simulink model "LQR_bloques_SS_LQR_cascada_PID_controller_NonLinear"  (R2023a)
settings: Solver=VariableStepAuto  StartTime=0.0  StopTime=t_sim  RelTol=1e-1
undefined symbols (not defined in the file): A, A_model, A_motor, B, B_mag0, B_model2, B_motor, C_model2, C_motor, D_motor, DeltaH_error_Gain, Error_ref_Gain, Gamma, I, J, K3_2, K4_2, K_gamma, Ke, Kt, La, Mgt_power_Gain, n_cal, omegaZ_inicial, R_mgt, Ra, RW_omega_max, RW_power_Gain, T_ext, T_max, T_max_mgt
libraries: simulink_extras x7, matrix_library x5, vrlib x2, slpidlib x2, aerolibutil x1, simulink x1
(part 1 of 2)
settings Model: Creator=Personal  LastModifiedBy=Personal
settings SolverCC: ZeroCrossAlgorithm=Adaptive
settings DebuggingCC: MaskedZcDiagnostic=none  IgnoredZcDiagnostic=none

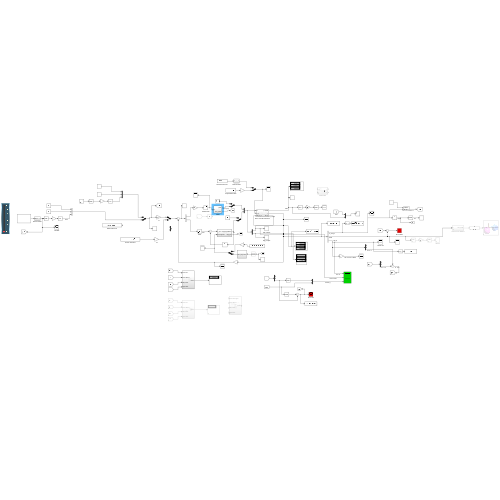
[thumbnail: Simulink's stored preview of the top-level diagram]
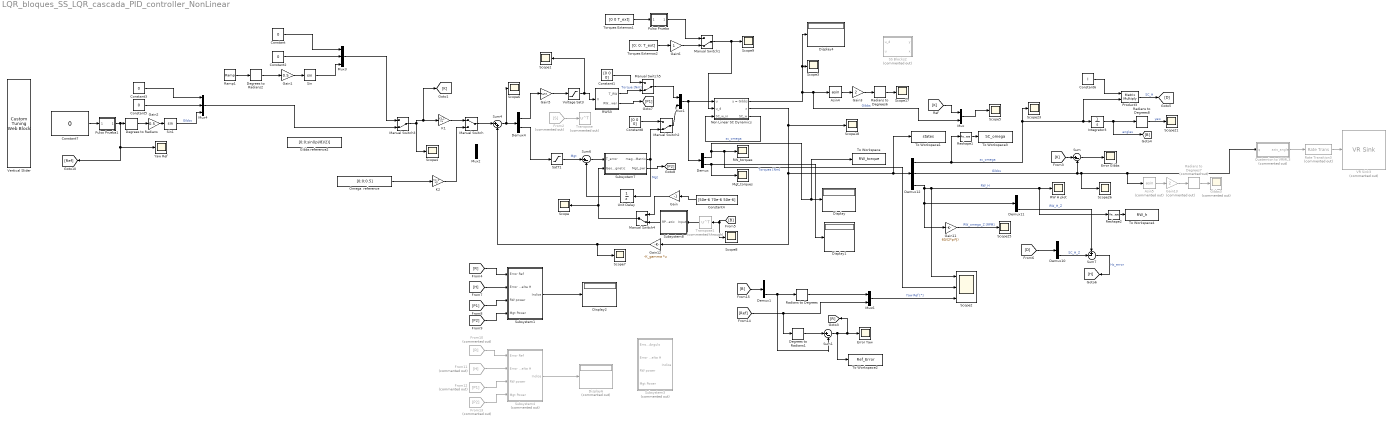
== system LQR_bloques_SS_LQR_cascada_PID_controller_NonLinear ==
  Asin4 : Trigonometry  Operator=asin
  Asin5 : Trigonometry  Commented=on  Operator=asin
  Constant{,2..3,5,7} (5 alike) : Constant  Value=0
  Constant1 : Constant  Value=[0 0 0]
  Constant4 : Constant  Value=[50e-6 70e-6 50e-6]
  Constant6 : Constant  Value=I
  Constant8 : Constant  Value=[0 0 0]
  Degrees to Radians : simulink_extras/Transformations/Degrees to Radians
  Degrees to Radians1 : simulink_extras/Transformations/Degrees to Radians
  Degrees to Radians2 : simulink_extras/Transformations/Degrees to Radians
  Demux : Demux  Outputs=2
  Demux{1,10..12} (4 alike) : Demux  Outputs=3
  Demux4 : Demux  Outputs=2
  Display{,1..2,4} (4 alike) : Display
  Display6 : Display  Commented=on
  Error Gibbs : Scope
  Error Yaw : Scope
  From10 : From  Commented=on  GotoTag=R
  From11 : From  Commented=on  GotoTag=H
  From12 : From  Commented=on  GotoTag=P1
  From13 : From  Commented=on  GotoTag=P2
  From2 : From  Commented=on  GotoTag=S
  Gain : Gain  Gain=-1
  Gain1 : Gain  Gain=0.5
  Gain11 : Gain  Gain=60/(2*pi*J)
  Gain12 : Gain  Gain=-K_gamma  Multiplication=Matrix(K*u)
  Gain13 : Gain  Commented=on  Gain=2
  Gain2 : Gain  Gain=0.5
  Gain3 : Gain  Gain=2
  Gain5 : Gain  Gain=Ra/Kt
  Gain6 : Gain
  Gibbs reference2 : Constant  Value=[0;0;sin((pi/8)/2)]  VectorParams1D=off
  Gibbs3 : Scope  Commented=on
  Integrator3 : Integrator  InitialCondition=[0;0;0]
  K1 : Gain  Gain=K3_2  Multiplication=Matrix(K*u)
  K2 : Gain  Gain=K4_2  Multiplication=Matrix(K*u)
  Manual Switch : ManualSwitch
  Manual Switch{1..5} (5 alike) : ManualSwitch  CurrentSetting=0
  Mgt_torques : Scope
  Mux{,1..2,6} (4 alike) : Mux  Inputs=2
  Mux3 : Mux  Inputs=3
  Mux4 : Mux  Inputs=3
  Non Linear SC Dynamics : Subsystem
  Omega  reference : Constant  Value=[0;0;0.5]
  Product3 : Product  Multiplication=Matrix(*)
  Pulso Prueba : Subsystem
  Pulso Prueba1 : Subsystem
  Quaternion to VRML3 : Subsystem  Commented=on
  RW H plot : Scope
  RWS3 : Subsystem
  RW_torques : Scope
  Radians to Degrees : simulink_extras/Transformations/Radians to Degrees
  Radians to Degrees6 : simulink_extras/Transformations/Radians to Degrees
  Radians to Degrees7 : simulink_extras/Transformations/Radians to Degrees  Commented=on
  Radians to Degrees8 : simulink_extras/Transformations/Radians to Degrees
  Ramp1 : simulink/Sources/Ramp  slope=0.5  start=0  InitialOutput=0
  Rate Transition3 : RateTransition  Commented=on
  Reshape1 : Reshape
  Reshape2 : Reshape
  SS Blocks2 : Subsystem  Commented=on
  SatT1 : Saturate  UpperLimit=T_max_mgt  LowerLimit=-T_max_mgt
  Scope{,1,3..9,17..18,21,23,25..26} (15 alike) : Scope
  Scope2 : Scope  NumInputPorts=3
  Sin : Trigonometry
  Sin1 : Trigonometry
  Subsystem1 : Subsystem
  Subsystem3 : Subsystem  Commented=on
  Subsystem4 : Subsystem  Commented=on
  Subsystem7 : Subsystem
  Subsystem8 : Subsystem
  Sum : Sum  Inputs=|+-
  Sum1 : Sum  Inputs=|+-
  Sum4 : Sum  Inputs=|++
  Sum6 : Sum  Inputs=|+-
  Sum7 : Sum  Inputs=+-|
  To Workspace : ToWorkspace  VariableName=RW_torque  SaveFormat=Structure With Time  SampleTime=-1
  To Workspace1 : ToWorkspace  VariableName=states  SaveFormat=Structure With Time  SampleTime=-1
  To Workspace2 : ToWorkspace  VariableName=Ref_Error  SaveFormat=Structure With Time  SampleTime=-1
  To Workspace3 : ToWorkspace  VariableName=SC_omega  SaveFormat=Structure With Time  SampleTime=-1
  To Workspace4 : ToWorkspace  VariableName=RW_h  SaveFormat=Structure With Time  SampleTime=-1
  Torques Externos1 : Constant  Value=[0 0 T_ext]
  Torques Externos2 : Constant  Value=[0; 0; T_ext]
  Transpose : Math  Commented=on  Operator=transpose
  Transpose1 : Math  Commented=through  Operator=transpose
  Unit Delay : UnitDelay  SampleTime=-1  HasFrameUpgradeWarning=on
  VR Sink3 : vrlib/VR Sink  Commented=on  InstantiateOnLoad=on  SampleTime=0.1  ViewEnable=on  RemoteChange=off  RemoteView=off  FieldsWritten=STLB_Transform.rotation.4.1.1.double  WorldFileName=EscenarioCubeSat.x3d  AutoView=off  VideoDimensions=[]  AllowVariableSize=off
  Vertical Slider : CustomTuningWebBlock  LabelPosition=Hide  ShowInitialText=on  Configuration="{\"components\":[{\"name\":\"LinearScaleComponent\",\"settings\":{\"bounds\":{\"max\":360,\"min\":0,\"tickInterval\":\"auto\"},\"internalTickHeightScaleFactor\":0.5,\"labelColor\":[255,255,200],\"labelFont\":{\"font\":\"Arial\",\"fontSize\":12},\"labelOffset\":0.05,\"labelTransparency\":1,\"needleImage\":{\"size\":[596,842],\"src\":\"data:image\\/svg+xml;base64,PD94bWwgdmVyc2lvbj0iMS4wIiBlbmNvZGluZz0idXRmLTgiPz4NCjwhLS0gR2VuZXJhdG9yOiBBZG9iZSBJbGx1c3RyYXRvciAyNS4wLjAsIFNWRyBFeHBvcnQgUGx1Zy1JbiAuIFNWRyBWZXJzaW9uOiA2LjAwIEJ1aWxkIDApICAtLT4NCjxzdmcgdmVyc2lvbj0iMS4xIg0KCSBpZD0ic3ZnOCIgeG1sbnM6Y2M9Imh0dHA6Ly9jcmVhdGl2ZWNvbW1vbnMub3JnL25zIyIgeG1sbnM6ZGM9Imh0dHA6Ly9wdXJsLm9yZy9kYy9lbGVtZW50cy8xLjEvIiB4bWxuczppbmtzY2FwZT0iaHR0cDovL3d3dy5pbmtzY2FwZS5vcmcvbmFtZXNw ...(+2420 chars)\",\"srcOrientation\":\"horizontal\"},\"needleOffset\":[0.0642123287671233,-0.8044596912521441],\"needleSize\":{\"height\":0.07668067226890757,\"width\":0.4337797619047619},\"position\":[0.03623949579831933,0.2829861111111111,0.6088789682539683,0.9196428571428571],\"referencePoint\":\"auto\",\"scaleColors\":[],\"scaleColorsSize\":0.2,\"scaleDirection\":\"BT\",\"showLabels\":1,\"showMinorTicks\":0,\"showSpanLine\":1,\"showTicks\":1,\"tickColor\":[252,252,197],\"tickTransparency\":1,\"valueBarColor\":[0,114,189],\"valueBarOffset\":-0.27,\"valueBarSize\":0.1,\"valueBarTransparency\":1}},{\"name\":\"BackgroundImageComponent\",\"settings\":{\"image\":{\"size\":[380,101],\"src\":\"data:image\\/svg+xml;base64,PHN2ZyB4bWxucz0iaHR0cDovL3d3dy53My5vcmcvMjAwMC9zdmciIHhtbG5zOnhsaW5rPSJodHRwOi8vd3d3LnczLm9yZy8xOTk5L3hsaW5rIiB2aWV3Qm94PSIwIDAgMzgwIDEwMSI+PGRlZnM+PHN0eWxlPi5jbHMtMXtmaWxsOiMwMDJiNDI7fS5jbHMtMntmaWxsOiM0MjcwODI7fS5jbHMtM3tmaWxsOnVybCgjcmFkaWFsLWdyYWRpZW50KTt9LmNscy00e2ZpbGw6I2M4YzhjODtzdHJva2U6IzAwMDt9PC9zdHlsZT48cmFkaWFsR3JhZGllbnQgaWQ9InJhZGlhbC1ncmFkaWVudCIgY3g9IjE5MCIgY3k9IjUwLjUiIHI9IjI2OS4yMSIgZ3JhZGllbnRVbml0cz0idXNlclNwYWNlT25Vc2UiPjxzdG9wIG9mZnNldD0iMC4wMSIgc3RvcC1jb2xvcj0iIzNlNGY1OCIvPjxzdG9wIG9mZnNldD0iMC4wNiIgc3RvcC1jb2xvcj0iIzQ0NTc2MSIvPjxzdG9wIG9mZnNldD0iMC4xNSIgc3RvcC1jb2xvcj0iIzU1NmE3NiIvPjxzdG9wIG9mZnNldD0iMC4yNSIgc3RvcC1jb2xvcj0iIzZkODg5NSIvPjxzdG9wIG9mZnNldD0iMC4zOCIgc3RvcC1jb2xvcj0iIzhmYjJjMyIvPjxzdG9wIG9mZnNldD0iMC41MiIgc3RvcC1jb2xvcj0iI2I2ZTRmYSIvPjxzdG9wIG9mZnNldD0iMSIgc3RvcC1jb2xvcj0iIzE1NDY1NyIvPjwvcmFkaWFsR3JhZGllbnQ+PC9kZWZzPjxnIGlkPSJmcmFtZSI+PGcgaWQ9IkxheWVyXzIiIGRhdGEtbmFtZT0iTGF5ZXIgMiI+PGcgaWQ9IkxheWVyXzEtMiIgZGF0YS1uYW1lPSJMYXllciAxLTIiPjxyZWN0IGlkPSJyZWN0MTAzNiIgY2xhc3M9ImNscy0xIiB4PSIxMSIgeT0iMTEiIHdpZHRoPSIzNTgiIGhlaWdodD0iNzkiLz48cGF0aCBpZD0icGF0aDEwMzgiIGNsYXNzPSJjbHMtMiIgZD0iTTgsOFY5M0gzNzJWOFpNMzY5LDkwSDExVjExSDM2OVoiLz48cGF0aCBpZD0icGF0aDEwNDAiIGNsYXNzPSJjbHMtMyIgZD0iTTAsMFYxMDFIMzgwVjBaTTM3Miw5M0g4VjhIMzcyWiIvPjwvZz48L2c+PC9nPjxnIGlkPSJ0cmFjayI+PHBhdGggaWQ9InJlY3QxNjExIiBjbGFzcz0iY2xzLTQiIGQ9Ik0zMy4zNywyNi41OUgzNDYuNjNjNCwwLDcuMjUsMi42LDcuMjUsNS44MWgwYzAsMy4yMS0zLjI1LDUuODItNy4yNSw1LjgySDMzLjM3Yy00LDAtNy4yNS0yLjYxLTcuMjUtNS44MmgwQzI2LjEyLDI5LjE5LDI5LjM3LDI2LjU5LDMzLjM3LDI2LjU5WiIvPjwvZz48L3N2Zz4=\",\"srcOrientation\":\"horizontal\"},\"position\":[0,0,1,1],\"scaleMode\":\"0\"}},{\"name\":\"ForegroundImageComponent\",\"settings\":{\"image\":{\"size\":[0,0],\"src\":\"default\",\"srcOrientation\":[]},\"isForeground\":1,\"position\":[0,0,1,1],\"scaleMode\":\"0\"}}],\"settings\":{\"BindingType\":\"param\",\"aspectRatio\":3.7777777777777777,\"backgroundColor\":[0,0,0,\"1\"],\"backgroundOffset\":0,\"backgroundOpacity\":1,\"fixedAspectRatio\":\"on\",\"foregroundColor\":[252,252,196],\"orientation\":\"vertical\",\"showBackgroundColor\":false,\"value\":0,\"version\":\"R2023a\"},\"type\":\"LinearGauge\"}"
  Voltage Sat3 : Saturate  UpperLimit=6  LowerLimit=-6
  Yaw Ref : Scope
  wires:
  K1/1 -> Manual Switch/1
  Mux1/1 -> Non Linear SC Dynamics/1(u), Demux/1
  Gain3/1 -> Radians to Degrees6/1
  Non Linear SC Dynamics/1(y = Gibbs) -> Display4/1, Scope3/1, Mux/2, Asin4/1  "Gibbs"
  Asin4/1 -> Gain3/1
  Radians to Degrees6/1 -> Scope17/1
  Demux/1 -> To Workspace/1, Display/1, Scope2/2, RW_torques/1  "Torques [Nm]"
  Demux/2 -> Display1/1, Mgt_torques/1
  Voltage Sat3/1 -> Scope1/1, RWS3/1(V)
  Gain5/1 -> Voltage Sat3/1
  SatT1/1 -> Sum6/1  "Mgt"
  Sum6/1 -> Subsystem7/1(T_error)
  Manual Switch4/1 -> Subsystem7/2(Geomagnetic), Scope/1
  Demux4/1 -> Gain5/1
  Demux4/2 -> SatT1/1
  Gain12/1 -> Scope7/1, Sum4/2
  Sum4/1 -> Scope6/1, Demux4/1
  Subsystem7/1(magTorqueMatrix) -> Unit Delay/1, Manual Switch2/2  "Mgt"
  RWS3/1(T_RW) -> Manual Switch5/2  "Torque [Nm]"
  Constant4/1 -> Gain/1
  Subsystem8/1(RPY_Magnetic) -> Manual Switch4/2
  Transpose1/1 -> Subsystem8/1(Input)
  Gain/1 -> Manual Switch4/1
  [D] -> Demux10/1
  Non Linear SC Dynamics/2(x) -> Gain12/1, To Workspace1/1, Demux12/1, Scope18/1
  Radians to Degrees7/1 -> Gibbs3/1
  Demux10/3 -> Sum7/2  "SC_H_Z"
  Radians to Degrees8/1 -> Scope21/1  "yaw"
  Demux11/3 -> Sum7/1  "RW_H_Z"
  Rate Transition3/1 -> VR Sink3/1
  Quaternion to VRML3/1(axis_angle) -> Rate Transition3/1
  Gain13/1 -> Radians to Degrees7/1
  Product3/1 -> [D]  "SC_H"
  Integrator3/1 -> [B], Radians to Degrees8/1  "angles"
  Gain11/1 -> Scope25/1  "RW_omega_Z [RPM]"
  Demux12/2 -> Asin5/1, Quaternion to VRML3/1(q), Scope26/1, Sum/2  "Gibbs"
  Sum7/1 -> [H]  "Hz_error"
  Asin5/1 -> Gain13/1
  Constant6/1 -> Product3/1
  Demux12/3 -> Scope2/1, Reshape2/1, RW H plot/1, Gain11/1, Demux11/1  "RW_H"
  Demux12/1 -> Integrator3/1, Product3/2, Scope23/1, Reshape1/1  "sc_omega"
  [B] -> Scope8/1, Transpose1/1
  Unit Delay/1 -> Sum6/2
  Omega  reference/1 -> K2/1
  Manual Switch/1 -> Sum4/1
  K2/1 -> Manual Switch/2
  Torques Externos2/1 -> Gain6/1
  Manual Switch2/1 -> Mux1/2
  Manual Switch3/1 -> Scope4/1, K1/1, [K]
  Mux/1 -> Scope5/1
  [K] -> Mux/1
  Manual Switch5/1 -> Mux1/1
  Constant1/1 -> Manual Switch5/1
  Non Linear SC Dynamics/3(SC_w) -> Non Linear SC Dynamics/3(SC_w_in)  "sc_omega"
  Manual Switch1/1 -> Scope9/1, Non Linear SC Dynamics/2(u_d)
  From2/1 -> Transpose/1
  Constant8/1 -> Manual Switch2/1
  [K] -> Sum/1
  Sum/1 -> Error Gibbs/1
  RWS3/2(RW_power) -> [P1]
  Subsystem7/2(Mgt_pwr) -> [P2]
  Ramp1/1 -> Degrees to Radians2/1
  Gain1/1 -> Sin/1
  Constant/1 -> Mux3/1
  Constant2/1 -> Mux3/2
  Mux3/1 -> Manual Switch3/1
  Sin/1 -> Mux3/3
  Mux4/1 -> Manual Switch3/2
  Constant5/1 -> Mux4/2
  Constant3/1 -> Mux4/1
  Gain2/1 -> Sin1/1
  Constant7/1 -> Pulso Prueba1/1(Ref in)
  Sin1/1 -> Mux4/3  "Gibbs"
  Degrees to Radians2/1 -> Gain1/1
  [H] -> Subsystem1/2(Error delta H)
  [R] -> Subsystem1/1(Error Ref)
  [P1] -> Subsystem1/3(RW power)
  [P2] -> Subsystem1/4(Mgt Power)
  Subsystem1/1(Indice) -> Display2/1
  Torques Externos1/1 -> Pulso Prueba/1(In1)
  Pulso Prueba/1(Out1) -> Manual Switch1/1
  Gain6/1 -> Manual Switch1/2
  Radians to Degrees/1 -> Mux6/1
  Subsystem4/1(Indice) -> Display6/1
  From13/1 -> Subsystem4/4(Mgt Power)
  From12/1 -> Subsystem4/3(RW power)
  From11/1 -> Subsystem4/2(Error delta H)
  From10/1 -> Subsystem4/1(Error Ref)
  [Ref] -> Degrees to Radians1/1, Mux6/2
  Mux6/1 -> Scope2/3  "Yaw Ref [°]"
  Pulso Prueba1/1(Out1) -> [Ref], Yaw Ref/1, Degrees to Radians/1
  Degrees to Radians/1 -> Gain2/1
  Sum1/1 -> To Workspace2/1, [R], Error Yaw/1
  Degrees to Radians1/1 -> Sum1/1
  Demux1/3 -> Sum1/2, Radians to Degrees/1
  [B] -> Demux1/1
  Reshape1/1 -> To Workspace3/1
  Reshape2/1 -> To Workspace4/1

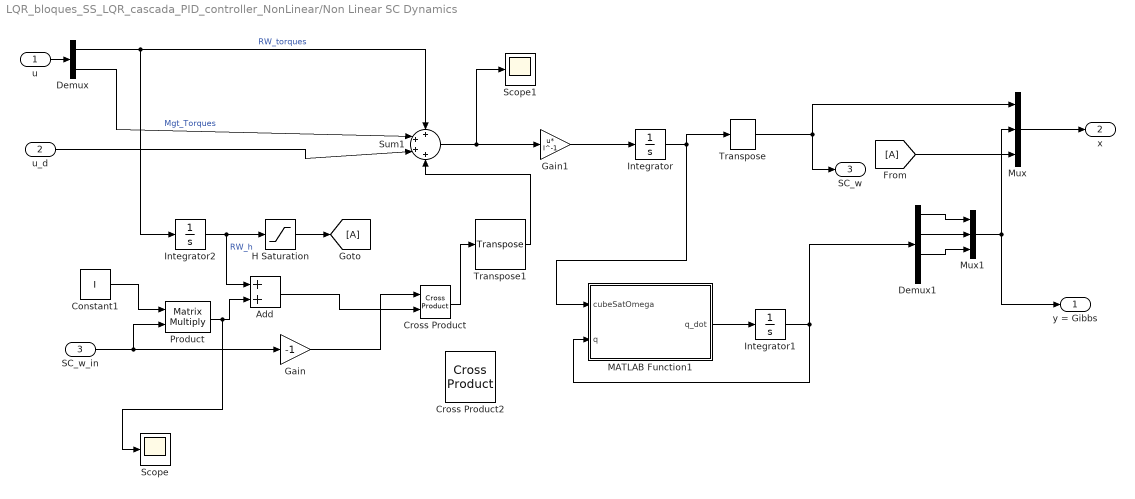
== system LQR_bloques_SS_LQR_cascada_PID_controller_NonLinear/Non Linear SC Dynamics ==
  u : Inport
  u_d : Inport  Port=2
  SC_w_in : Inport  Port=3
  Add : Sum
  Constant1 : Constant  Value=I
  Cross Product : vrlib/Utilities/Cross Product
  Cross Product2 : matrix_library/Cross Product
  Demux : Demux  Outputs=2
  Demux1 : Demux
  From : From
  Gain : Gain  Gain=-1
  Gain1 : Gain  Gain=I^-1  Multiplication=Matrix(u*K)
  Goto : Goto
  H Saturation : Saturate  UpperLimit=J*RW_omega_max  LowerLimit=-J*RW_omega_max
  Integrator : Integrator  InitialCondition=[0 0 omegaZ_inicial]
  Integrator1 : Integrator  InitialCondition=[0 0 0 1]
  Integrator2 : Integrator  InitialCondition=[0 0 0]
  MATLAB Function1 : MATLAB Function  TreatAsAtomicUnit=on
  Mux : Mux  Inputs=3
  Mux1 : Mux  Inputs=3
  Product : Product  Multiplication=Matrix(*)
  Scope : Scope
  Scope1 : Scope
  Sum1 : Sum  Inputs=++++
  Transpose : matrix_library/Transpose
  Transpose1 : matrix_library/Transpose
  y = Gibbs : Outport
  x : Outport  Port=2
  SC_w : Outport  Port=3
  wires:
  Demux/1 -> Integrator2/1, Sum1/1  "RW_torques"
  u_d/1 -> Sum1/3
  Integrator1/1 -> Demux1/1, MATLAB Function1/2(q)
  Constant1/1 -> Product/1
  Product/1 -> Scope/1, Add/2
  Integrator2/1 -> H Saturation/1, Add/1  "RW_h"
  Gain/1 -> Cross Product/1
  Add/1 -> Cross Product/2
  Cross Product/1 -> Transpose1/1
  Sum1/1 -> Scope1/1, Gain1/1
  Gain1/1 -> Integrator/1
  Integrator/1 -> MATLAB Function1/1(cubeSatOmega), Transpose/1
  MATLAB Function1/1(q_dot) -> Integrator1/1
  SC_w_in/1 -> Product/2, Gain/1
  Transpose/1 -> SC_w/1, Mux/1
  Transpose1/1 -> Sum1/4
  Demux/2 -> Sum1/2  "Mgt_Torques"
  u/1 -> Demux/1
  Mux/1 -> x/1
  Demux1/1 -> Mux1/1
  Demux1/2 -> Mux1/2
  Demux1/3 -> Mux1/3
  Mux1/1 -> Mux/2, y = Gibbs/1
  From/1 -> Mux/3
  H Saturation/1 -> Goto/1

== system LQR_bloques_SS_LQR_cascada_PID_controller_NonLinear/Pulso Prueba ==
  In1 : Inport
  Product1 : Product
  Scope5 : Scope
  Step2 : Step  Time=500  SampleTime=0
  Step3 : Step  Time=6000  After=-2  SampleTime=0
  Sum : Sum  Inputs=|++
  Out1 : Outport
  wires:
  Step2/1 -> Sum/1
  Step3/1 -> Sum/2
  In1/1 -> Product1/2
  Sum/1 -> Product1/1, Scope5/1
  Product1/1 -> Out1/1

== system LQR_bloques_SS_LQR_cascada_PID_controller_NonLinear/Pulso Prueba1 ==
  Ref in : Inport
  Gain : Gain  Gain=-1
  Product1 : Product
  Scope5 : Scope
  Step2 : Step  Time=2000  SampleTime=0
  Step3 : Step  Time=14000  After=2  SampleTime=0
  Sum : Sum  Inputs=|++
  Out1 : Outport
  wires:
  Product1/1 -> Out1/1
  Sum/1 -> Scope5/1, Product1/1
  Ref in/1 -> Product1/2
  Step3/1 -> Gain/1
  Step2/1 -> Sum/1
  Gain/1 -> Sum/2

== system LQR_bloques_SS_LQR_cascada_PID_controller_NonLinear/Quaternion to VRML3 ==
  q : Inport
  Asin1 : Trigonometry  Operator=asin
  Constant : Constant  Value=pi/2
  Demux : Demux  Outputs=3
  "Flip 180 deg, rotate 90" : Constant  Value=[0 0.2 0 0]
  Gain2 : Gain  Gain=2
  Mux : Mux
  Quaternion Multiplication : aerolibutil/Quaternion Multiplication
  Saturation : Saturate
  Selector1 : Selector  InputPortWidth=4  IndexOptions=Index vector (dialog)  Indices=[2 3 1 4]  OutputSizes=1
  Sum : Sum  Inputs=|+-
  axis_angle : Outport  VectorParamsAs1DForOutWhenUnconnected=off
  wires:
  Constant/1 -> Sum/1
  Saturation/1 -> Asin1/1
  Asin1/1 -> Gain2/1
  Demux/3 -> Mux/3, Saturation/1
  Gain2/1 -> Mux/4
  Selector1/1 -> axis_angle/1
  Mux/1 -> Selector1/1
  Demux/1 -> Mux/1
  q/1 -> Demux/1
  "Flip 180 deg, rotate 90"/1 -> Quaternion Multiplication/2
  Demux/2 -> Mux/2

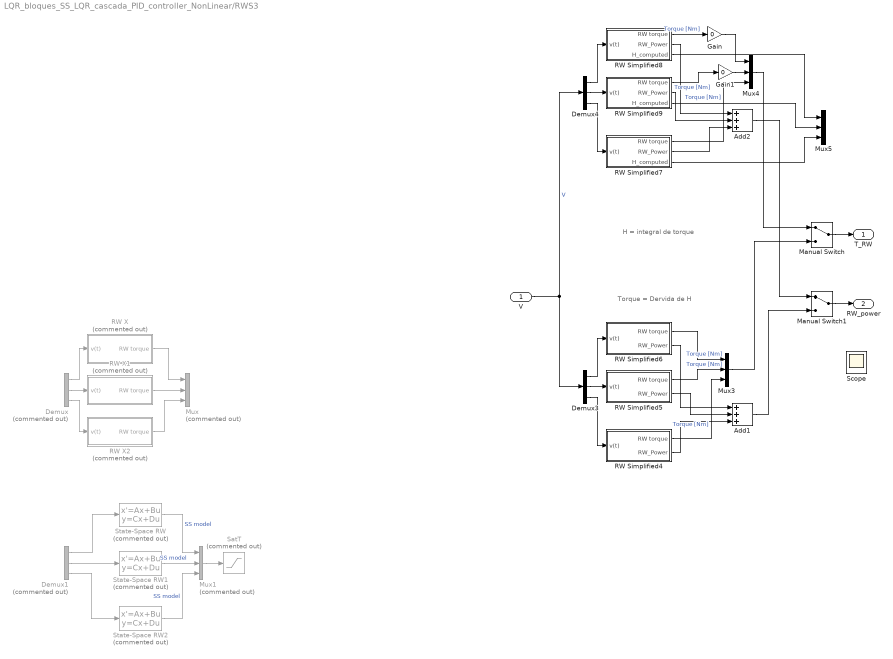
== system LQR_bloques_SS_LQR_cascada_PID_controller_NonLinear/RWS3 ==
  note: Torque = Dervida de H
  note: H = integral de torque
  V : Inport
  Add1 : Sum  Inputs=+++
  Add2 : Sum  Inputs=+++
  Demux : Demux  Commented=on  Outputs=3
  Demux1 : Demux  Commented=on  Outputs=3
  Demux3 : Demux  Outputs=3
  Demux4 : Demux  Outputs=3
  Gain : Gain  Gain=0
  Gain1 : Gain  Gain=0
  Manual Switch : ManualSwitch
  Manual Switch1 : ManualSwitch
  Mux : Mux  Commented=on  Inputs=3
  Mux1 : Mux  Commented=on  Inputs=3
  Mux3 : Mux  Inputs=3
  Mux4 : Mux  Inputs=3
  Mux5 : Mux  Inputs=3
  RW Simplified4 : Subsystem
  RW Simplified5 : Subsystem
  RW Simplified6 : Subsystem
  RW Simplified7 : Subsystem
  RW Simplified8 : Subsystem
  RW Simplified9 : Subsystem
  RW X : Subsystem  Commented=on
  RW X1 : Subsystem  Commented=on
  RW X2 : Subsystem  Commented=on
  SatT : Saturate  Commented=on  UpperLimit=T_max  LowerLimit=-T_max
  Scope : Scope
  State-Space RW : StateSpace  Commented=on  A=A_motor  B=B_motor  C=C_motor  D=D_motor  InitialCondition=0
  State-Space RW1 : StateSpace  Commented=on  A=A_motor  B=B_motor  C=C_motor  D=D_motor  InitialCondition=0
  State-Space RW2 : StateSpace  Commented=on  A=A_motor  B=B_motor  C=C_motor  D=D_motor  InitialCondition=0
  T_RW : Outport
  RW_power : Outport  Port=2
  wires:
  Demux/1 -> RW X/1(v(t))
  Demux/3 -> RW X2/1(v(t))
  Demux/2 -> RW X1/1(v(t))
  RW X2/1(RW torque) -> Mux/3
  Demux1/1 -> State-Space RW/1
  Demux1/2 -> State-Space RW1/1
  Demux1/3 -> State-Space RW2/1
  State-Space RW1/1 -> Mux1/2  "SS model"
  State-Space RW/1 -> Mux1/1  "SS model"
  State-Space RW2/1 -> Mux1/3  "SS model"
  Mux1/1 -> SatT/1
  Manual Switch/1 -> T_RW/1
  RW X/1(RW torque) -> Mux/1
  RW X1/1(RW torque) -> Mux/2
  RW Simplified6/2(RW_Power) -> Add1/1
  RW Simplified5/2(RW_Power) -> Add1/2
  Mux3/1 -> Manual Switch/2
  RW Simplified4/1(RW torque) -> Mux3/3  "Torque [Nm]"
  RW Simplified5/1(RW torque) -> Mux3/2  "Torque [Nm]"
  RW Simplified6/1(RW torque) -> Mux3/1  "Torque [Nm]"
  Demux3/3 -> RW Simplified4/1(v(t))
  Demux3/2 -> RW Simplified5/1(v(t))
  Demux3/1 -> RW Simplified6/1(v(t))
  RW Simplified4/2(RW_Power) -> Add1/3
  Add1/1 -> Manual Switch1/2
  Manual Switch1/1 -> RW_power/1
  RW Simplified9/3(H_computed) -> Mux5/2
  Gain1/1 -> Mux4/2
  Demux4/1 -> RW Simplified8/1(v(t))
  Gain/1 -> Mux4/1
  Add2/1 -> Manual Switch1/1
  RW Simplified7/1(RW torque) -> Mux4/3  "Torque [Nm]"
  RW Simplified7/3(H_computed) -> Mux5/3
  RW Simplified8/2(RW_Power) -> Add2/1
  RW Simplified9/1(RW torque) -> Gain1/1  "Torque [Nm]"
  Mux4/1 -> Manual Switch/1
  Demux4/2 -> RW Simplified9/1(v(t))
  RW Simplified9/2(RW_Power) -> Add2/2
  Demux4/3 -> RW Simplified7/1(v(t))
  V/1 -> Demux4/1, Demux3/1  "V"
  RW Simplified8/3(H_computed) -> Mux5/1
  RW Simplified7/2(RW_Power) -> Add2/3
  RW Simplified8/1(RW torque) -> Gain/1  "Torque [Nm]"

== system LQR_bloques_SS_LQR_cascada_PID_controller_NonLinear/SS Blocks2 ==
  u_d : Inport
  u : Inport  Port=2
  A : Gain  Gain=A_model  Multiplication=Matrix(K*u)
  B : Gain  Gain=B_model2  Multiplication=Matrix(K*u)
  C : Gain  Gain=C_model2  Multiplication=Matrix(K*u)
  Gamma : Gain  Gain=Gamma  Multiplication=Matrix(K*u)
  Integrator : Integrator  InitialCondition=zeros(9,1)
  Sum : Sum  Inputs=+++
  y : Outport
  x : Outport  Port=2
  wires:
  B/1 -> Sum/2
  u/1 -> B/1
  Sum/1 -> Integrator/1  "x_dot"
  A/1 -> Sum/3
  C/1 -> y/1
  Integrator/1 -> C/1, x/1, A/1
  u_d/1 -> Gamma/1
  Gamma/1 -> Sum/1

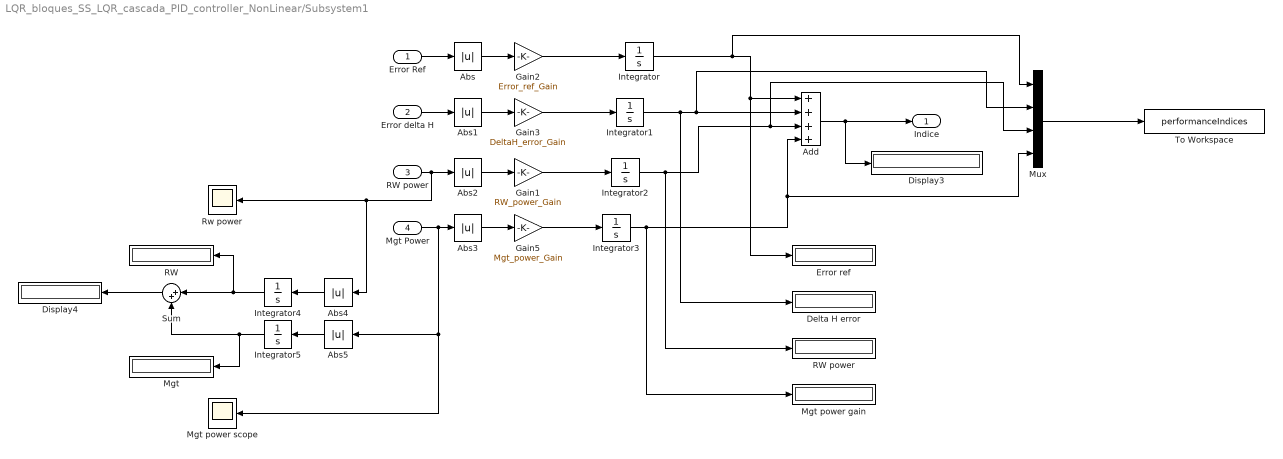
== system LQR_bloques_SS_LQR_cascada_PID_controller_NonLinear/Subsystem1 ==
  Error Ref : Inport
  Error delta H : Inport  Port=2
  RW power : Inport  Port=3
  Mgt Power : Inport  Port=4
  Abs{,1..5} (6 alike) : Abs  SaturateOnIntegerOverflow=off
  Add : Sum  Inputs=++++
  Delta H error : Display
  Display3 : Display
  Display4 : Display
  Error ref : Display
  Gain1 : Gain  Gain=RW_power_Gain
  Gain2 : Gain  Gain=Error_ref_Gain
  Gain3 : Gain  Gain=DeltaH_error_Gain
  Gain5 : Gain  Gain=Mgt_power_Gain
  Integrator{,1..5} (6 alike) : Integrator
  Mgt : Display
  Mgt power gain : Display
  Mgt power scope : Scope
  Mux : Mux
  RW : Display
  "RW power " : Display
  Rw power : Scope
  Sum : Sum  Inputs=|++
  To Workspace : ToWorkspace  VariableName=performanceIndices  SaveFormat=Structure With Time  SampleTime=-1
  Indice : Outport
  wires:
  Gain1/1 -> Integrator2/1
  Abs1/1 -> Gain3/1
  Abs/1 -> Gain2/1
  Abs2/1 -> Gain1/1
  Abs3/1 -> Gain5/1
  Gain3/1 -> Integrator1/1
  Gain5/1 -> Integrator3/1
  RW power/1 -> Abs4/1, Rw power/1, Abs2/1
  Error delta H/1 -> Abs1/1
  Gain2/1 -> Integrator/1
  Integrator1/1 -> Delta H error/1, Mux/2, Add/2
  Integrator2/1 -> Mux/3, Add/3, "RW power "/1
  Integrator3/1 -> Add/4, Mux/4, Mgt power gain/1
  Add/1 -> Indice/1, Display3/1
  Integrator4/1 -> RW/1, Sum/1
  Integrator5/1 -> Mgt/1, Sum/2
  Sum/1 -> Display4/1
  Mgt Power/1 -> Abs5/1, Mgt power scope/1, Abs3/1
  Abs4/1 -> Integrator4/1
  Abs5/1 -> Integrator5/1
  Error Ref/1 -> Abs/1
  Mux/1 -> To Workspace/1
  Integrator/1 -> Mux/1, Add/1, Error ref/1

== system LQR_bloques_SS_LQR_cascada_PID_controller_NonLinear/Subsystem3 ==
  Error Ref Angulo : Inport
  Error delta H : Inport  Port=2
  RW power : Inport  Port=3
  Mgt Power : Inport  Port=4
  Abs{,1..3} (4 alike) : Abs  SaturateOnIntegerOverflow=off
  Add : Sum  Inputs=++++
  Clock : Clock
  Display{1..7} (7 alike) : Display
  Gain1 : Gain  Gain=0.8
  Gain2 : Gain
  Gain3 : Gain
  Gain5 : Gain  Gain=0.6
  Integrator : Integrator
  Product1 : Product
  Product2 : Product
  Indice : Outport
  wires:
  Integrator/1 -> Indice/1, Display3/1
  Error Ref Angulo/1 -> Abs/1
  Gain2/1 -> Product2/1
  Gain1/1 -> Display2/1, Add/3
  Abs1/1 -> Gain3/1
  Abs/1 -> Gain2/1
  Abs2/1 -> Gain1/1
  Abs3/1 -> Gain5/1
  Product1/1 -> Display6/1, Add/2
  Add/1 -> Display5/1, Integrator/1
  Gain5/1 -> Display1/1, Add/4
  RW power/1 -> Abs2/1
  Mgt Power/1 -> Abs3/1
  Gain3/1 -> Product1/1
  Error delta H/1 -> Abs1/1
  Clock/1 -> Product2/2, Product1/2, Display4/1
  Product2/1 -> Display7/1, Add/1

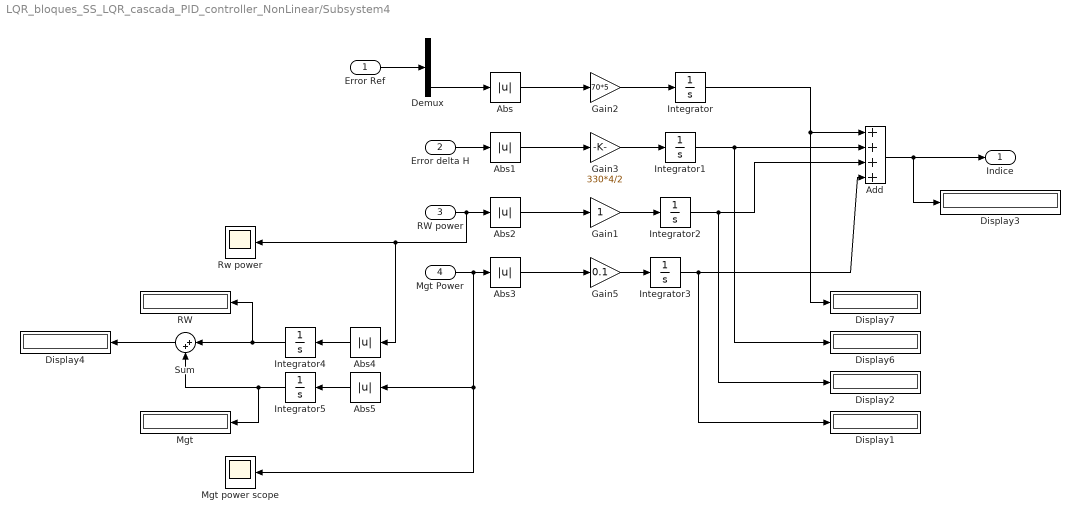
== system LQR_bloques_SS_LQR_cascada_PID_controller_NonLinear/Subsystem4 ==
  Error Ref : Inport
  Error delta H : Inport  Port=2
  RW power : Inport  Port=3
  Mgt Power : Inport  Port=4
  Abs{,1..5} (6 alike) : Abs  SaturateOnIntegerOverflow=off
  Add : Sum  Inputs=++++
  Demux : Demux  Outputs=3
  Display{1..4,6..7} (6 alike) : Display
  Gain1 : Gain
  Gain2 : Gain  Gain=70*5
  Gain3 : Gain  Gain=330*4/2
  Gain5 : Gain  Gain=0.1
  Integrator{,1..5} (6 alike) : Integrator
  Mgt : Display
  Mgt power scope : Scope
  RW : Display
  Rw power : Scope
  Sum : Sum  Inputs=|++
  Indice : Outport
  wires:
  Demux/3 -> Abs/1
  Abs5/1 -> Integrator5/1
  Abs4/1 -> Integrator4/1
  Mgt Power/1 -> Abs3/1, Mgt power scope/1, Abs5/1
  Sum/1 -> Display4/1
  Integrator5/1 -> Sum/2, Mgt/1
  Integrator4/1 -> Sum/1, RW/1
  Add/1 -> Display3/1, Indice/1
  Integrator3/1 -> Display1/1, Add/4
  Integrator2/1 -> Display2/1, Add/3
  Integrator1/1 -> Add/2, Display6/1
  Integrator/1 -> Display7/1, Add/1
  Gain2/1 -> Integrator/1
  Error delta H/1 -> Abs1/1
  RW power/1 -> Abs2/1, Rw power/1, Abs4/1
  Gain5/1 -> Integrator3/1
  Gain3/1 -> Integrator1/1
  Abs3/1 -> Gain5/1
  Abs2/1 -> Gain1/1
  Abs/1 -> Gain2/1
  Abs1/1 -> Gain3/1
  Gain1/1 -> Integrator2/1
  Error Ref/1 -> Demux/1

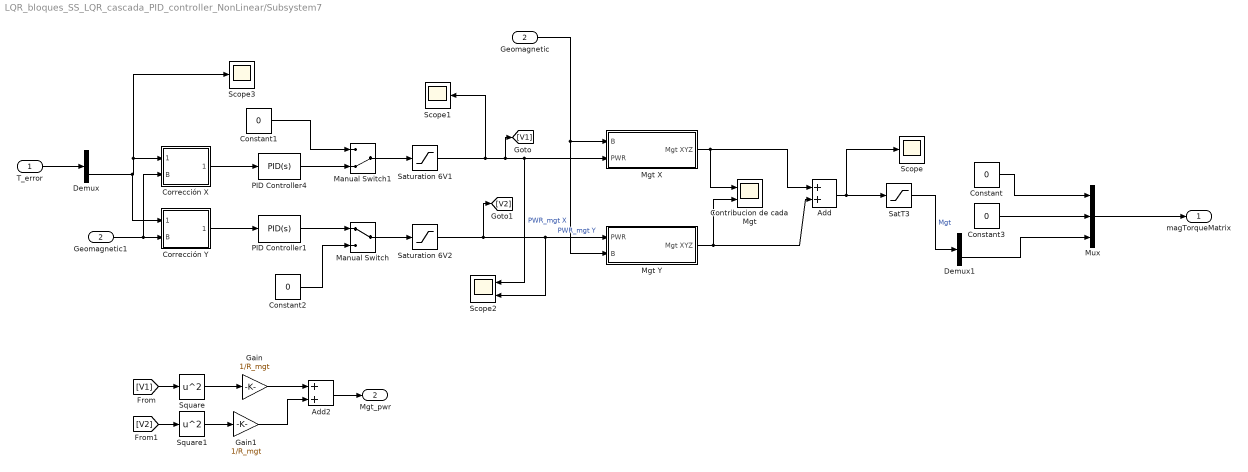
== system LQR_bloques_SS_LQR_cascada_PID_controller_NonLinear/Subsystem7 ==
  T_error : Inport
  Geomagnetic : Inport  Port=2
  Add : Sum
  Add2 : Sum
  Constant{,1..3} (4 alike) : Constant  Value=0
  Contribucion de cada Mgt : Scope  NumInputPorts=2
  Corrección X : MATLAB Function  TreatAsAtomicUnit=on
  Corrección Y : MATLAB Function  TreatAsAtomicUnit=on
  Demux : Demux  Outputs=3
  Demux1 : Demux  Outputs=3
  Gain : Gain  Gain=1/R_mgt
  Gain1 : Gain  Gain=1/R_mgt
  Geomagnetic1 : InportShadow  Port=2
  Manual Switch : ManualSwitch
  Manual Switch1 : ManualSwitch  CurrentSetting=0
  Mgt X : Subsystem
  Mgt Y : Subsystem
  Mux : Mux  Inputs=3
  PID Controller1 : slpidlib/PID Controller  Controller=PID  Form=Parallel  TimeDomain=Continuous-time  UseExternalTs=off  SampleTime=-1  IntegratorMethod=Forward Euler  FilterMethod=Forward Euler  ControllerParametersSource=internal  P=3739538.59240439  I=11683234637.8679  UseKiTs=off  D=-2886.42122409877  N=1295.56232513222  UseFilter=on  TunerSelectOption=Transfer Function Based (PID Tuner App)  InitialConditionSource=internal  InitialConditionForIntegrator=0  InitialConditionForFilter=0  DifferentiatorICPrevScaledInput=0  ExternalReset=none  TrackingMode=off  Kt=1  LimitOutput=on  SatLimitsSource=internal  UpperSaturationLimit=5  LowerSaturationLimit=-5  LinearizeAsGain=on  AntiWindupMode=clamping  Kb=1  LimitIntegrator=off  UpperIntegratorSaturationLimit=inf  LowerIntegratorSaturationLimit=-inf  POutMin=[]  POutMax=[]  IOutMin=[]  IOutMax=[]  DOutMin=[]  DOutMax=[]  NOutMin=[]  NOutMax=[]  SumOutMin=[]  SumOutMax=[]  SaturationOutMin=[]  SaturationOutMax=[]  PParamMin=[]  PParamMax=[]  IParamMin=[]  IParamMax=[]  DParamMin=[]  DParamMax=[]  NParamMin=[]  NParamMax=[]  KbParamMin=[]  KbParamMax=[]  KtParamMin=[]  KtParamMax=[]  KbOutMin=[]  KbOutMax=[]  KtOutMin=[]  KtOutMax=[]  IntegratorOutMin=[]  IntegratorOutMax=[]  FilterOutMin=[]  FilterOutMax=[]  SumI1OutMin=[]  SumI1OutMax=[]  SumI2OutMin=[]  SumI2OutMax=[]  SumI3OutMin=[]  SumI3OutMax=[]  SumI4OutMin=[]  SumI4OutMax=[]  SumDOutMin=[]  SumDOutMax=[]  DifferentiatorOutMin=[]  DifferentiatorOutMax=[]  FilterDiffOutCoefMin=[]  FilterDiffOutCoefMax=[]  ReciprocalOutMin=[]  ReciprocalOutMax=[]  SumDenOutMin=[]  SumDenOutMax=[]  SumNumOutMin=[]  SumNumOutMax=[]  DivideOutMin=[]  DivideOutMax=[]  UdiffTsProdOutMin=[]  UdiffTsProdOutMax=[]  NTsProdOutMin=[]  NTsProdOutMax=[]  UintegralTsProdOutMin=[]  UintegralTsProdOutMax=[]  UngainTsProdOutMin=[]  UngainTsProdOutMax=[]  ClampingZeroOutDataTypeStr=Inherit: Inherit via back propagation  ClampingZeroOutMin=[]  ClampingZeroOutMax=[]  FilterDenConstantOutDataTypeStr=Inherit: Inherit via back propagation  FilterDenConstantOutMin=[]  FilterDenConstantOutMax=[]  PCopyOutDataTypeStr=Inherit: Inherit via back propagation  PCopyOutMin=[]  PCopyOutMax=[]  NCopyOutDataTypeStr=Inherit: Inherit via back propagation  NCopyOutMin=[]  NCopyOutMax=[]  IntegratorContinuousStateAttributes=''  IntegratorStateMustResolveToSignalObject=off  IntegratorRTWStateStorageClass=Auto  FilterContinuousStateAttributes=''  FilterStateMustResolveToSignalObject=off  FilterRTWStateStorageClass=Auto  ParallelPVariant=InternalParameters  IdealPVariant=Disabled  IVariant=InternalParameters  DVariant=InternalParameters  IntegratorVariant=Continuous  SatVariant=Enabled  AWVariant=ContClampingParallel  PCopyVariant=Disabled  TRVariant=Disabled  FdbkBlocksVariant=Forward  IdealPFdbkVariant=Disabled  SatFdbkVariant=Disabled  DerivativeFilterVariant=ContFilter  NVariant=InternalParameters  NCopyVariant=Disabled  FilterICVariant=InternalICsFilter  IntegratorICVariant=InternalICs  ExternalResetVariant=Disabled  TRSumVariant=Passthrough  SumFdbkVariant=Disabled  SumVariant=Sum_PID  TsampFilterVariant=InternalTs  TsampNgainVariant=Passthrough  TsampIntegralVariant=Disabled_SignalSpec  ExternalSaturationOutDataTypeStr=Inherit: Same as second input
  PID Controller4 : slpidlib/PID Controller  Controller=PID  Form=Parallel  TimeDomain=Continuous-time  UseExternalTs=off  SampleTime=-1  IntegratorMethod=Forward Euler  FilterMethod=Forward Euler  ControllerParametersSource=internal  P=3739538.59240439  I=11683234637.8679  UseKiTs=off  D=-2886.42122409877  N=1295.56232513222  UseFilter=on  TunerSelectOption=Transfer Function Based (PID Tuner App)  InitialConditionSource=internal  InitialConditionForIntegrator=0  InitialConditionForFilter=0  DifferentiatorICPrevScaledInput=0  ExternalReset=none  TrackingMode=off  Kt=1  LimitOutput=on  SatLimitsSource=internal  UpperSaturationLimit=5  LowerSaturationLimit=-5  LinearizeAsGain=on  AntiWindupMode=clamping  Kb=1  LimitIntegrator=off  UpperIntegratorSaturationLimit=inf  LowerIntegratorSaturationLimit=-inf  POutMin=[]  POutMax=[]  IOutMin=[]  IOutMax=[]  DOutMin=[]  DOutMax=[]  NOutMin=[]  NOutMax=[]  SumOutMin=[]  SumOutMax=[]  SaturationOutMin=[]  SaturationOutMax=[]  PParamMin=[]  PParamMax=[]  IParamMin=[]  IParamMax=[]  DParamMin=[]  DParamMax=[]  NParamMin=[]  NParamMax=[]  KbParamMin=[]  KbParamMax=[]  KtParamMin=[]  KtParamMax=[]  KbOutMin=[]  KbOutMax=[]  KtOutMin=[]  KtOutMax=[]  IntegratorOutMin=[]  IntegratorOutMax=[]  FilterOutMin=[]  FilterOutMax=[]  SumI1OutMin=[]  SumI1OutMax=[]  SumI2OutMin=[]  SumI2OutMax=[]  SumI3OutMin=[]  SumI3OutMax=[]  SumI4OutMin=[]  SumI4OutMax=[]  SumDOutMin=[]  SumDOutMax=[]  DifferentiatorOutMin=[]  DifferentiatorOutMax=[]  FilterDiffOutCoefMin=[]  FilterDiffOutCoefMax=[]  ReciprocalOutMin=[]  ReciprocalOutMax=[]  SumDenOutMin=[]  SumDenOutMax=[]  SumNumOutMin=[]  SumNumOutMax=[]  DivideOutMin=[]  DivideOutMax=[]  UdiffTsProdOutMin=[]  UdiffTsProdOutMax=[]  NTsProdOutMin=[]  NTsProdOutMax=[]  UintegralTsProdOutMin=[]  UintegralTsProdOutMax=[]  UngainTsProdOutMin=[]  UngainTsProdOutMax=[]  ClampingZeroOutDataTypeStr=Inherit: Inherit via back propagation  ClampingZeroOutMin=[]  ClampingZeroOutMax=[]  FilterDenConstantOutDataTypeStr=Inherit: Inherit via back propagation  FilterDenConstantOutMin=[]  FilterDenConstantOutMax=[]  PCopyOutDataTypeStr=Inherit: Inherit via back propagation  PCopyOutMin=[]  PCopyOutMax=[]  NCopyOutDataTypeStr=Inherit: Inherit via back propagation  NCopyOutMin=[]  NCopyOutMax=[]  IntegratorContinuousStateAttributes=''  IntegratorStateMustResolveToSignalObject=off  IntegratorRTWStateStorageClass=Auto  FilterContinuousStateAttributes=''  FilterStateMustResolveToSignalObject=off  FilterRTWStateStorageClass=Auto  ParallelPVariant=InternalParameters  IdealPVariant=Disabled  IVariant=InternalParameters  DVariant=InternalParameters  IntegratorVariant=Continuous  SatVariant=Enabled  AWVariant=ContClampingParallel  PCopyVariant=Disabled  TRVariant=Disabled  FdbkBlocksVariant=Forward  IdealPFdbkVariant=Disabled  SatFdbkVariant=Disabled  DerivativeFilterVariant=ContFilter  NVariant=InternalParameters  NCopyVariant=Disabled  FilterICVariant=InternalICsFilter  IntegratorICVariant=InternalICs  ExternalResetVariant=Disabled  TRSumVariant=Passthrough  SumFdbkVariant=Disabled  SumVariant=Sum_PID  TsampFilterVariant=InternalTs  TsampNgainVariant=Passthrough  TsampIntegralVariant=Disabled_SignalSpec  ExternalSaturationOutDataTypeStr=Inherit: Same as second input
  SatT3 : Saturate  UpperLimit=T_max_mgt  LowerLimit=-T_max_mgt
  Saturation 6V1 : Saturate  UpperLimit=5  LowerLimit=-5
  Saturation 6V2 : Saturate  UpperLimit=5  LowerLimit=-5
  Scope : Scope
  Scope1 : Scope
  Scope2 : Scope  NumInputPorts=2
  Scope3 : Scope
  Square : Math  Operator=square
  Square1 : Math  Operator=square
  magTorqueMatrix : Outport
  Mgt_pwr : Outport  Port=2
  wires:
  PID Controller4/1 -> Manual Switch1/2
  Saturation 6V1/1 -> [V1], Scope2/1, Mgt X/2(PWR), Scope1/1  "PWR_mgt X"
  Geomagnetic/1 -> Mgt Y/2(B), Mgt X/1(B)
  Manual Switch/1 -> Saturation 6V2/1
  Constant1/1 -> Manual Switch1/1
  Manual Switch1/1 -> Saturation 6V1/1
  Saturation 6V2/1 -> [V2], Scope2/2, Mgt Y/1(PWR)  "PWR_mgt Y"
  Add/1 -> SatT3/1, Scope/1
  T_error/1 -> Demux/1
  Mgt X/1(Mgt XYZ) -> Contribucion de cada Mgt/1, Add/1
  Mgt Y/1(Mgt XYZ) -> Add/2, Contribucion de cada Mgt/2
  Constant2/1 -> Manual Switch/2
  Demux/3 -> Corrección Y/1("T_error "), Corrección X/1("T_error "), Scope3/1
  SatT3/1 -> Demux1/1  "Mgt"
  Corrección X/1(T_error) -> PID Controller4/1
  Geomagnetic1/1 -> Corrección X/2(B), Corrección Y/2(B)
  Demux1/3 -> Mux/3
  Constant/1 -> Mux/1
  Constant3/1 -> Mux/2
  Mux/1 -> magTorqueMatrix/1
  Corrección Y/1(T_error) -> PID Controller1/1
  PID Controller1/1 -> Manual Switch/1
  Square1/1 -> Gain1/1
  [V1] -> Square/1
  Gain1/1 -> Add2/2
  Square/1 -> Gain/1
  Gain/1 -> Add2/1
  Add2/1 -> Mgt_pwr/1
  [V2] -> Square1/1

== system LQR_bloques_SS_LQR_cascada_PID_controller_NonLinear/Subsystem8 ==
  Input : Inport
  Clock : Clock
  Constant1 : Constant  Value=B_mag0
  Extract B : MATLAB Function  TreatAsAtomicUnit=on
  MATLAB Function : MATLAB Function  TreatAsAtomicUnit=on
  Scope1 : Scope
  Scope8 : Scope
  Zero-Order Hold : ZeroOrderHold  SampleTime=-1
  RPY_Magnetic : Outport
  wires:
  Constant1/1 -> Extract B/1(B_cal)
  Extract B/1(XYZ_Magnetic) -> MATLAB Function/1(NEDMagnetic), Scope8/1
  Input/1 -> MATLAB Function/2(RPY)
  Zero-Order Hold/1 -> Scope1/1, Extract B/2(time)
  MATLAB Function/1(RPY_Magnetic) -> RPY_Magnetic/1
  Clock/1 -> Zero-Order Hold/1

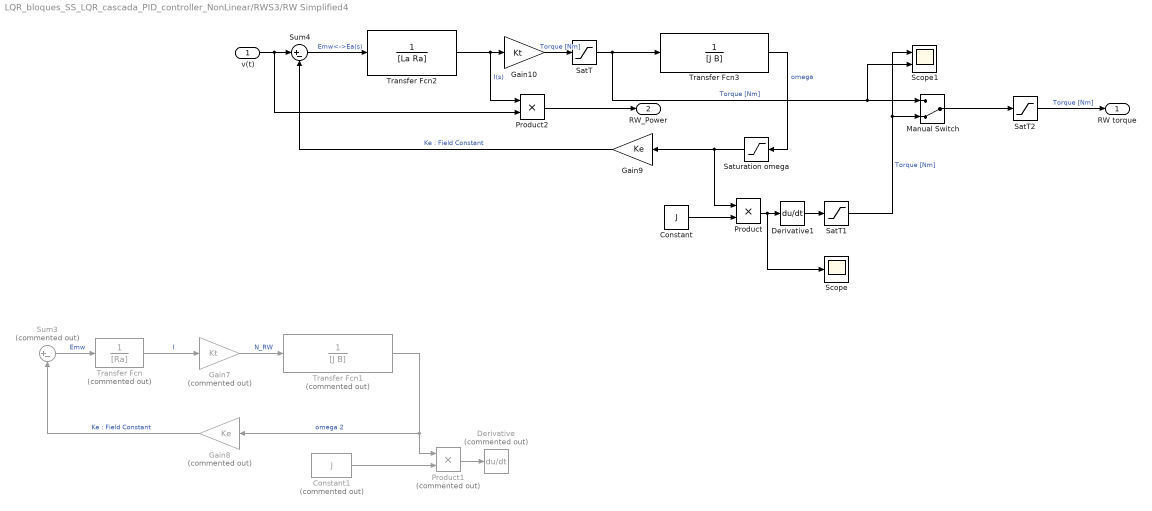
== system LQR_bloques_SS_LQR_cascada_PID_controller_NonLinear/RWS3/RW Simplified4 ==
  v(t) : Inport
  Constant : Constant  Value=J
  Constant1 : Constant  Commented=on  Value=J
  Derivative : Derivative  Commented=on
  Derivative1 : Derivative
  Gain10 : Gain  Gain=Kt
  Gain7 : Gain  Commented=on  Gain=Kt
  Gain8 : Gain  Commented=on  Gain=Ke
  Gain9 : Gain  Gain=Ke
  Manual Switch : ManualSwitch  CurrentSetting=0
  Product : Product
  Product1 : Product  Commented=on
  Product2 : Product
  SatT : Saturate  UpperLimit=T_max  LowerLimit=-T_max
  SatT1 : Saturate  UpperLimit=T_max  LowerLimit=-T_max
  SatT2 : Saturate  UpperLimit=T_max  LowerLimit=-T_max
  Saturation omega : Saturate  UpperLimit=RW_omega_max  LowerLimit=-RW_omega_max
  Scope : Scope
  Scope1 : Scope  NumInputPorts=2
  Sum3 : Sum  Commented=on  Inputs=|+-
  Sum4 : Sum  Inputs=|+-
  Transfer Fcn : TransferFcn  Commented=on  Denominator=[Ra]
  Transfer Fcn1 : TransferFcn  Commented=on  Denominator=[J B]
  Transfer Fcn2 : TransferFcn  Denominator=[La Ra]
  Transfer Fcn3 : TransferFcn  Denominator=[J B]
  RW torque : Outport  VectorParamsAs1DForOutWhenUnconnected=off
  RW_Power : Outport  Port=2  VectorParamsAs1DForOutWhenUnconnected=off
  wires:
  SatT2/1 -> RW torque/1  "Torque [Nm]"
  Saturation omega/1 -> Gain9/1, Product/1
  Manual Switch/1 -> SatT2/1
  SatT1/1 -> Manual Switch/2, Scope1/1  "Torque [Nm]"
  Derivative1/1 -> SatT1/1
  Product/1 -> Derivative1/1, Scope/1
  Product2/1 -> RW_Power/1
  SatT/1 -> Transfer Fcn3/1, Scope1/2, Manual Switch/1  "Torque [Nm]"
  Gain10/1 -> SatT/1  "Torque [Nm]"
  Gain8/1 -> Sum3/2  "Ke : Field Constant"
  Transfer Fcn/1 -> Gain7/1  "I"
  Sum3/1 -> Transfer Fcn/1  "Emw"
  Gain7/1 -> Transfer Fcn1/1  "N_RW"
  Transfer Fcn1/1 -> Gain8/1, Product1/1  "omega 2"
  Constant1/1 -> Product1/2
  Product1/1 -> Derivative/1
  v(t)/1 -> Sum4/1, Product2/2
  Constant/1 -> Product/2
  Transfer Fcn3/1 -> Saturation omega/1  "omega"
  Gain9/1 -> Sum4/2  "Ke : Field Constant"
  Sum4/1 -> Transfer Fcn2/1  "Emw<->Ea(s)"
  Transfer Fcn2/1 -> Gain10/1, Product2/1  "I(s)"

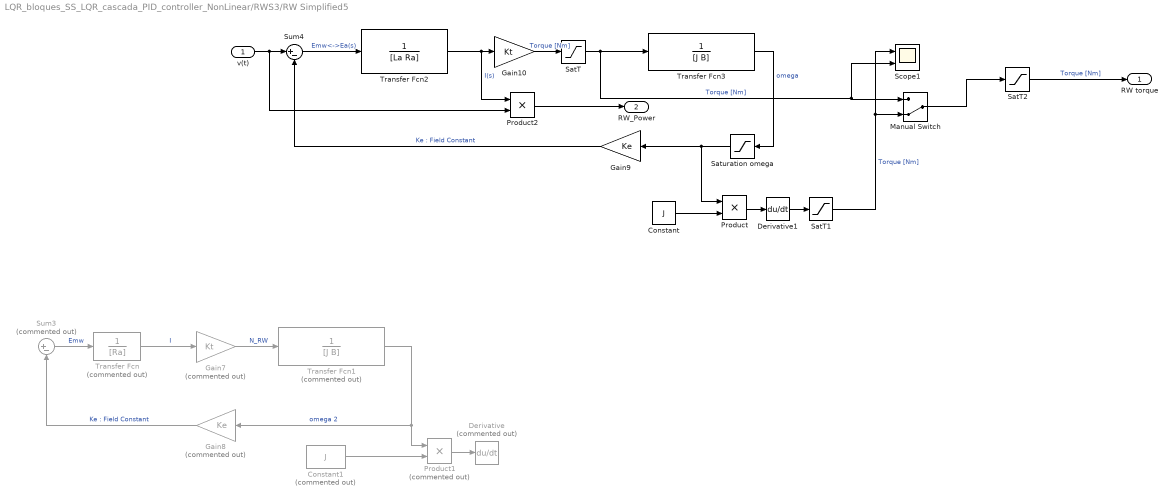
== system LQR_bloques_SS_LQR_cascada_PID_controller_NonLinear/RWS3/RW Simplified5 ==
  v(t) : Inport
  Constant : Constant  Value=J
  Constant1 : Constant  Commented=on  Value=J
  Derivative : Derivative  Commented=on
  Derivative1 : Derivative
  Gain10 : Gain  Gain=Kt
  Gain7 : Gain  Commented=on  Gain=Kt
  Gain8 : Gain  Commented=on  Gain=Ke
  Gain9 : Gain  Gain=Ke
  Manual Switch : ManualSwitch  CurrentSetting=0
  Product : Product
  Product1 : Product  Commented=on
  Product2 : Product
  SatT : Saturate  UpperLimit=T_max  LowerLimit=-T_max
  SatT1 : Saturate  UpperLimit=T_max  LowerLimit=-T_max
  SatT2 : Saturate  UpperLimit=T_max  LowerLimit=-T_max
  Saturation omega : Saturate  UpperLimit=RW_omega_max  LowerLimit=-RW_omega_max
  Scope1 : Scope  NumInputPorts=2
  Sum3 : Sum  Commented=on  Inputs=|+-
  Sum4 : Sum  Inputs=|+-
  Transfer Fcn : TransferFcn  Commented=on  Denominator=[Ra]
  Transfer Fcn1 : TransferFcn  Commented=on  Denominator=[J B]
  Transfer Fcn2 : TransferFcn  Denominator=[La Ra]
  Transfer Fcn3 : TransferFcn  Denominator=[J B]
  RW torque : Outport  VectorParamsAs1DForOutWhenUnconnected=off
  RW_Power : Outport  Port=2  VectorParamsAs1DForOutWhenUnconnected=off
  wires:
  Transfer Fcn2/1 -> Product2/1, Gain10/1  "I(s)"
  Sum4/1 -> Transfer Fcn2/1  "Emw<->Ea(s)"
  Gain9/1 -> Sum4/2  "Ke : Field Constant"
  Transfer Fcn3/1 -> Saturation omega/1  "omega"
  Constant/1 -> Product/2
  v(t)/1 -> Product2/2, Sum4/1
  Product1/1 -> Derivative/1
  Constant1/1 -> Product1/2
  Transfer Fcn1/1 -> Product1/1, Gain8/1  "omega 2"
  Gain7/1 -> Transfer Fcn1/1  "N_RW"
  Sum3/1 -> Transfer Fcn/1  "Emw"
  Transfer Fcn/1 -> Gain7/1  "I"
  Gain8/1 -> Sum3/2  "Ke : Field Constant"
  Gain10/1 -> SatT/1  "Torque [Nm]"
  SatT/1 -> Manual Switch/1, Scope1/2, Transfer Fcn3/1  "Torque [Nm]"
  Product2/1 -> RW_Power/1
  Product/1 -> Derivative1/1
  Derivative1/1 -> SatT1/1
  SatT1/1 -> Scope1/1, Manual Switch/2  "Torque [Nm]"
  Manual Switch/1 -> SatT2/1
  Saturation omega/1 -> Product/1, Gain9/1
  SatT2/1 -> RW torque/1  "Torque [Nm]"

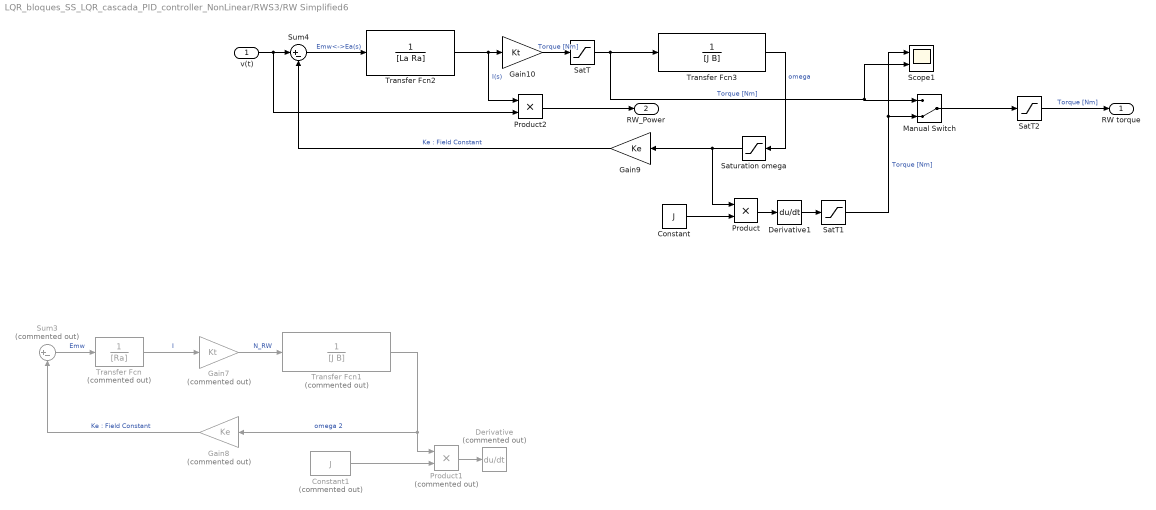
== system LQR_bloques_SS_LQR_cascada_PID_controller_NonLinear/RWS3/RW Simplified6 ==
  v(t) : Inport
  Constant : Constant  Value=J
  Constant1 : Constant  Commented=on  Value=J
  Derivative : Derivative  Commented=on
  Derivative1 : Derivative
  Gain10 : Gain  Gain=Kt
  Gain7 : Gain  Commented=on  Gain=Kt
  Gain8 : Gain  Commented=on  Gain=Ke
  Gain9 : Gain  Gain=Ke
  Manual Switch : ManualSwitch  CurrentSetting=0
  Product : Product
  Product1 : Product  Commented=on
  Product2 : Product
  SatT : Saturate  UpperLimit=T_max  LowerLimit=-T_max
  SatT1 : Saturate  UpperLimit=T_max  LowerLimit=-T_max
  SatT2 : Saturate  UpperLimit=T_max  LowerLimit=-T_max
  Saturation omega : Saturate  UpperLimit=RW_omega_max  LowerLimit=-RW_omega_max
  Scope1 : Scope  NumInputPorts=2
  Sum3 : Sum  Commented=on  Inputs=|+-
  Sum4 : Sum  Inputs=|+-
  Transfer Fcn : TransferFcn  Commented=on  Denominator=[Ra]
  Transfer Fcn1 : TransferFcn  Commented=on  Denominator=[J B]
  Transfer Fcn2 : TransferFcn  Denominator=[La Ra]
  Transfer Fcn3 : TransferFcn  Denominator=[J B]
  RW torque : Outport  VectorParamsAs1DForOutWhenUnconnected=off
  RW_Power : Outport  Port=2  VectorParamsAs1DForOutWhenUnconnected=off
  wires:
  SatT2/1 -> RW torque/1  "Torque [Nm]"
  Saturation omega/1 -> Gain9/1, Product/1
  Manual Switch/1 -> SatT2/1
  SatT1/1 -> Manual Switch/2, Scope1/1  "Torque [Nm]"
  Derivative1/1 -> SatT1/1
  Product/1 -> Derivative1/1
  Product2/1 -> RW_Power/1
  SatT/1 -> Transfer Fcn3/1, Scope1/2, Manual Switch/1  "Torque [Nm]"
  Gain10/1 -> SatT/1  "Torque [Nm]"
  Gain8/1 -> Sum3/2  "Ke : Field Constant"
  Transfer Fcn/1 -> Gain7/1  "I"
  Sum3/1 -> Transfer Fcn/1  "Emw"
  Gain7/1 -> Transfer Fcn1/1  "N_RW"
  Transfer Fcn1/1 -> Gain8/1, Product1/1  "omega 2"
  Constant1/1 -> Product1/2
  Product1/1 -> Derivative/1
  v(t)/1 -> Sum4/1, Product2/2
  Constant/1 -> Product/2
  Transfer Fcn3/1 -> Saturation omega/1  "omega"
  Gain9/1 -> Sum4/2  "Ke : Field Constant"
  Sum4/1 -> Transfer Fcn2/1  "Emw<->Ea(s)"
  Transfer Fcn2/1 -> Gain10/1, Product2/1  "I(s)"

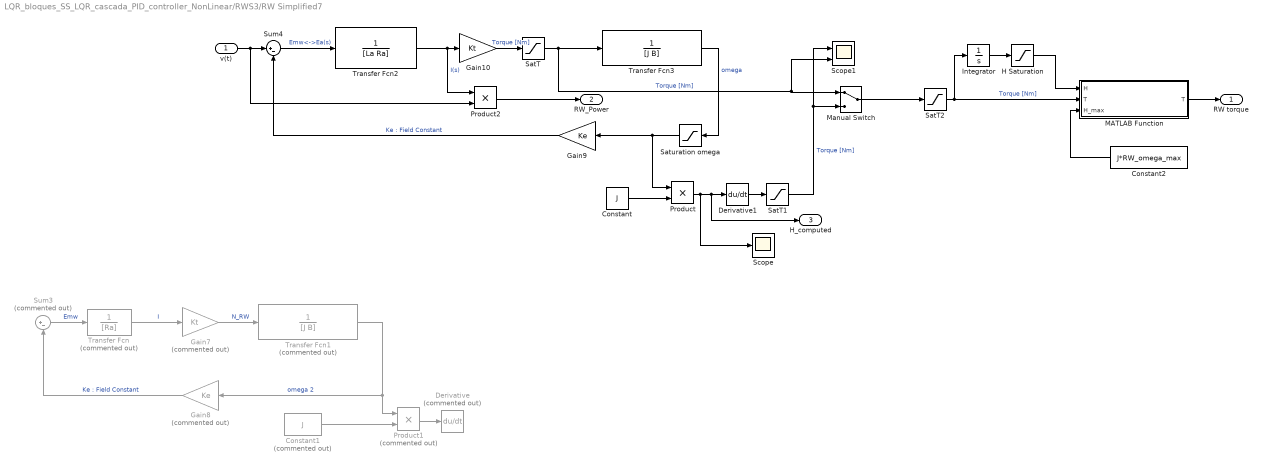
== system LQR_bloques_SS_LQR_cascada_PID_controller_NonLinear/RWS3/RW Simplified7 ==
  v(t) : Inport
  Constant : Constant  Value=J
  Constant1 : Constant  Commented=on  Value=J
  Constant2 : Constant  Value=J*RW_omega_max
  Derivative : Derivative  Commented=on
  Derivative1 : Derivative
  Gain10 : Gain  Gain=Kt
  Gain7 : Gain  Commented=on  Gain=Kt
  Gain8 : Gain  Commented=on  Gain=Ke
  Gain9 : Gain  Gain=Ke
  H Saturation : Saturate  UpperLimit=J*RW_omega_max  LowerLimit=-J*RW_omega_max
  Integrator : Integrator
  MATLAB Function : MATLAB Function  TreatAsAtomicUnit=on
  Manual Switch : ManualSwitch
  Product : Product
  Product1 : Product  Commented=on
  Product2 : Product
  SatT : Saturate  UpperLimit=T_max  LowerLimit=-T_max
  SatT1 : Saturate  UpperLimit=T_max  LowerLimit=-T_max
  SatT2 : Saturate  UpperLimit=T_max  LowerLimit=-T_max
  Saturation omega : Saturate  UpperLimit=RW_omega_max  LowerLimit=-RW_omega_max
  Scope : Scope
  Scope1 : Scope  NumInputPorts=2
  Sum3 : Sum  Commented=on  Inputs=|+-
  Sum4 : Sum  Inputs=|+-
  Transfer Fcn : TransferFcn  Commented=on  Denominator=[Ra]
  Transfer Fcn1 : TransferFcn  Commented=on  Denominator=[J B]
  Transfer Fcn2 : TransferFcn  Denominator=[La Ra]
  Transfer Fcn3 : TransferFcn  Denominator=[J B]
  RW torque : Outport  VectorParamsAs1DForOutWhenUnconnected=off
  RW_Power : Outport  Port=2  VectorParamsAs1DForOutWhenUnconnected=off
  H_computed : Outport  Port=3
  wires:
  Transfer Fcn2/1 -> Product2/1, Gain10/1  "I(s)"
  Sum4/1 -> Transfer Fcn2/1  "Emw<->Ea(s)"
  Gain9/1 -> Sum4/2  "Ke : Field Constant"
  Transfer Fcn3/1 -> Saturation omega/1  "omega"
  Constant/1 -> Product/2
  v(t)/1 -> Product2/2, Sum4/1
  Product1/1 -> Derivative/1
  Constant1/1 -> Product1/2
  Transfer Fcn1/1 -> Product1/1, Gain8/1  "omega 2"
  Gain7/1 -> Transfer Fcn1/1  "N_RW"
  Sum3/1 -> Transfer Fcn/1  "Emw"
  Transfer Fcn/1 -> Gain7/1  "I"
  Gain8/1 -> Sum3/2  "Ke : Field Constant"
  Gain10/1 -> SatT/1  "Torque [Nm]"
  SatT/1 -> Manual Switch/1, Scope1/2, Transfer Fcn3/1  "Torque [Nm]"
  Product2/1 -> RW_Power/1
  Product/1 -> Scope/1, H_computed/1, Derivative1/1
  Derivative1/1 -> SatT1/1
  SatT1/1 -> Scope1/1, Manual Switch/2  "Torque [Nm]"
  Manual Switch/1 -> SatT2/1
  Saturation omega/1 -> Product/1, Gain9/1
  SatT2/1 -> MATLAB Function/2("T "), Integrator/1  "Torque [Nm]"
  Integrator/1 -> H Saturation/1
  Constant2/1 -> MATLAB Function/3(H_max)
  H Saturation/1 -> MATLAB Function/1(H)
  MATLAB Function/1(T) -> RW torque/1

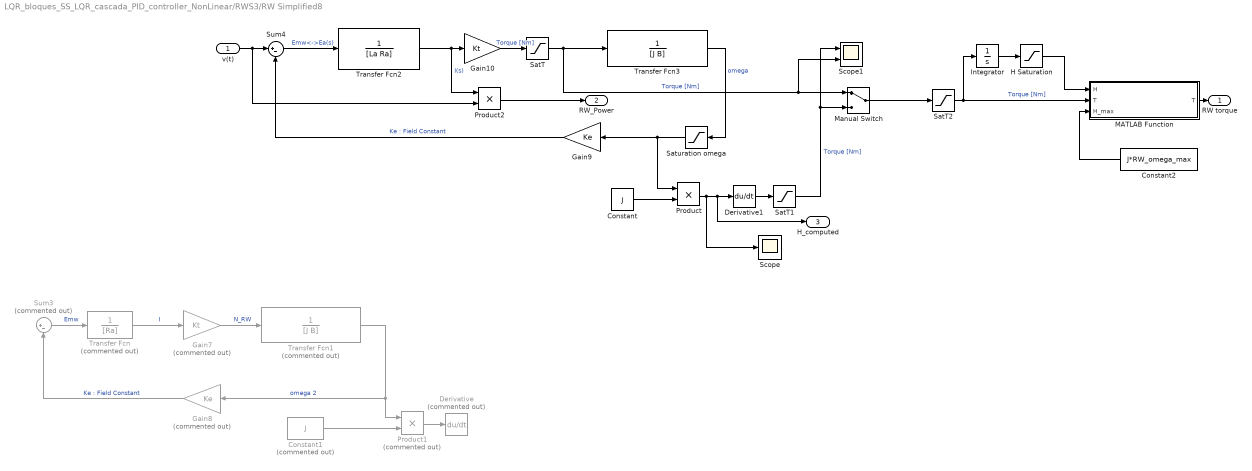
== system LQR_bloques_SS_LQR_cascada_PID_controller_NonLinear/RWS3/RW Simplified8 ==
  v(t) : Inport
  Constant : Constant  Value=J
  Constant1 : Constant  Commented=on  Value=J
  Constant2 : Constant  Value=J*RW_omega_max
  Derivative : Derivative  Commented=on
  Derivative1 : Derivative
  Gain10 : Gain  Gain=Kt
  Gain7 : Gain  Commented=on  Gain=Kt
  Gain8 : Gain  Commented=on  Gain=Ke
  Gain9 : Gain  Gain=Ke
  H Saturation : Saturate  UpperLimit=J*RW_omega_max  LowerLimit=-J*RW_omega_max
  Integrator : Integrator
  MATLAB Function : MATLAB Function  TreatAsAtomicUnit=on
  Manual Switch : ManualSwitch
  Product : Product
  Product1 : Product  Commented=on
  Product2 : Product
  SatT : Saturate  UpperLimit=T_max  LowerLimit=-T_max
  SatT1 : Saturate  UpperLimit=T_max  LowerLimit=-T_max
  SatT2 : Saturate  UpperLimit=T_max  LowerLimit=-T_max
  Saturation omega : Saturate  UpperLimit=RW_omega_max  LowerLimit=-RW_omega_max
  Scope : Scope
  Scope1 : Scope  NumInputPorts=2
  Sum3 : Sum  Commented=on  Inputs=|+-
  Sum4 : Sum  Inputs=|+-
  Transfer Fcn : TransferFcn  Commented=on  Denominator=[Ra]
  Transfer Fcn1 : TransferFcn  Commented=on  Denominator=[J B]
  Transfer Fcn2 : TransferFcn  Denominator=[La Ra]
  Transfer Fcn3 : TransferFcn  Denominator=[J B]
  RW torque : Outport  VectorParamsAs1DForOutWhenUnconnected=off
  RW_Power : Outport  Port=2  VectorParamsAs1DForOutWhenUnconnected=off
  H_computed : Outport  Port=3
  wires:
  Transfer Fcn2/1 -> Product2/1, Gain10/1  "I(s)"
  Sum4/1 -> Transfer Fcn2/1  "Emw<->Ea(s)"
  Gain9/1 -> Sum4/2  "Ke : Field Constant"
  Transfer Fcn3/1 -> Saturation omega/1  "omega"
  Constant/1 -> Product/2
  v(t)/1 -> Product2/2, Sum4/1
  Product1/1 -> Derivative/1
  Constant1/1 -> Product1/2
  Transfer Fcn1/1 -> Product1/1, Gain8/1  "omega 2"
  Gain7/1 -> Transfer Fcn1/1  "N_RW"
  Sum3/1 -> Transfer Fcn/1  "Emw"
  Transfer Fcn/1 -> Gain7/1  "I"
  Gain8/1 -> Sum3/2  "Ke : Field Constant"
  Gain10/1 -> SatT/1  "Torque [Nm]"
  SatT/1 -> Manual Switch/1, Scope1/2, Transfer Fcn3/1  "Torque [Nm]"
  Product2/1 -> RW_Power/1
  Product/1 -> Scope/1, H_computed/1, Derivative1/1
  Derivative1/1 -> SatT1/1
  SatT1/1 -> Scope1/1, Manual Switch/2  "Torque [Nm]"
  Manual Switch/1 -> SatT2/1
  Saturation omega/1 -> Product/1, Gain9/1
  SatT2/1 -> Integrator/1, MATLAB Function/2("T ")  "Torque [Nm]"
  Integrator/1 -> H Saturation/1
  Constant2/1 -> MATLAB Function/3(H_max)
  H Saturation/1 -> MATLAB Function/1(H)
  MATLAB Function/1(T) -> RW torque/1

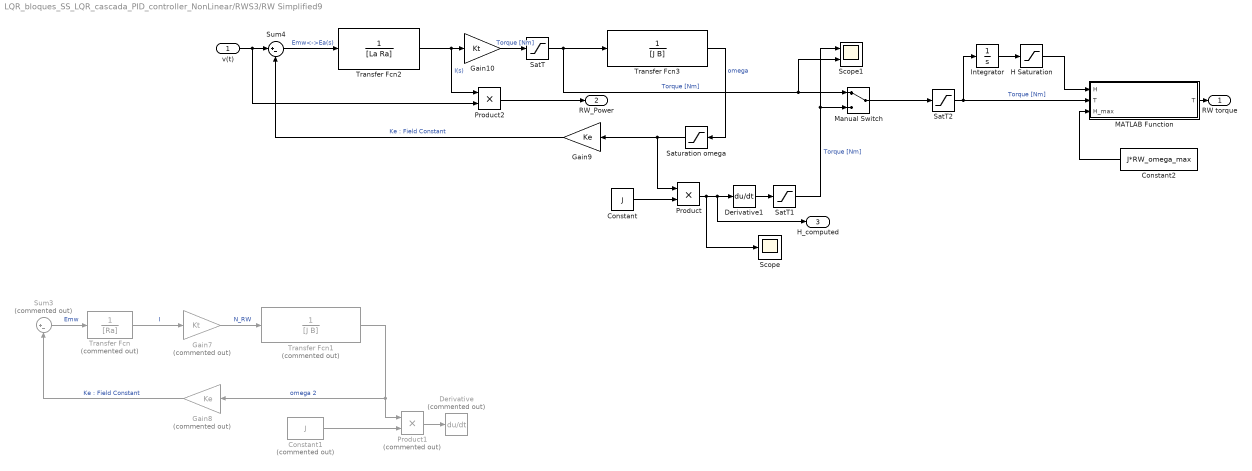
== system LQR_bloques_SS_LQR_cascada_PID_controller_NonLinear/RWS3/RW Simplified9 ==
  v(t) : Inport
  Constant : Constant  Value=J
  Constant1 : Constant  Commented=on  Value=J
  Constant2 : Constant  Value=J*RW_omega_max
  Derivative : Derivative  Commented=on
  Derivative1 : Derivative
  Gain10 : Gain  Gain=Kt
  Gain7 : Gain  Commented=on  Gain=Kt
  Gain8 : Gain  Commented=on  Gain=Ke
  Gain9 : Gain  Gain=Ke
  H Saturation : Saturate  UpperLimit=J*RW_omega_max  LowerLimit=-J*RW_omega_max
  Integrator : Integrator
  MATLAB Function : MATLAB Function  TreatAsAtomicUnit=on
  Manual Switch : ManualSwitch
  Product : Product
  Product1 : Product  Commented=on
  Product2 : Product
  SatT : Saturate  UpperLimit=T_max  LowerLimit=-T_max
  SatT1 : Saturate  UpperLimit=T_max  LowerLimit=-T_max
  SatT2 : Saturate  UpperLimit=T_max  LowerLimit=-T_max
  Saturation omega : Saturate  UpperLimit=RW_omega_max  LowerLimit=-RW_omega_max
  Scope : Scope
  Scope1 : Scope  NumInputPorts=2
  Sum3 : Sum  Commented=on  Inputs=|+-
  Sum4 : Sum  Inputs=|+-
  Transfer Fcn : TransferFcn  Commented=on  Denominator=[Ra]
  Transfer Fcn1 : TransferFcn  Commented=on  Denominator=[J B]
  Transfer Fcn2 : TransferFcn  Denominator=[La Ra]
  Transfer Fcn3 : TransferFcn  Denominator=[J B]
  RW torque : Outport  VectorParamsAs1DForOutWhenUnconnected=off
  RW_Power : Outport  Port=2  VectorParamsAs1DForOutWhenUnconnected=off
  H_computed : Outport  Port=3
  wires:
  MATLAB Function/1(T) -> RW torque/1
  H Saturation/1 -> MATLAB Function/1(H)
  Constant2/1 -> MATLAB Function/3(H_max)
  Integrator/1 -> H Saturation/1
  SatT2/1 -> MATLAB Function/2("T "), Integrator/1  "Torque [Nm]"
  Saturation omega/1 -> Gain9/1, Product/1
  Manual Switch/1 -> SatT2/1
  SatT1/1 -> Manual Switch/2, Scope1/1  "Torque [Nm]"
  Derivative1/1 -> SatT1/1
  Product/1 -> Derivative1/1, H_computed/1, Scope/1
  Product2/1 -> RW_Power/1
  SatT/1 -> Transfer Fcn3/1, Scope1/2, Manual Switch/1  "Torque [Nm]"
  Gain10/1 -> SatT/1  "Torque [Nm]"
  Gain8/1 -> Sum3/2  "Ke : Field Constant"
  Transfer Fcn/1 -> Gain7/1  "I"
  Sum3/1 -> Transfer Fcn/1  "Emw"
  Gain7/1 -> Transfer Fcn1/1  "N_RW"
  Transfer Fcn1/1 -> Gain8/1, Product1/1  "omega 2"
  Constant1/1 -> Product1/2
  Product1/1 -> Derivative/1
  v(t)/1 -> Sum4/1, Product2/2
  Constant/1 -> Product/2
  Transfer Fcn3/1 -> Saturation omega/1  "omega"
  Gain9/1 -> Sum4/2  "Ke : Field Constant"
  Sum4/1 -> Transfer Fcn2/1  "Emw<->Ea(s)"
  Transfer Fcn2/1 -> Gain10/1, Product2/1  "I(s)"
